simulink model "echo"  (R2020a)
settings: Solver=VariableStepAuto  StartTime=0.0  StopTime=10.0  RelTol=1e-3
libraries: dspspect3 x1, dspvision x1, dspobslib x1
settings Model: Creator=XPS 15  LastModifiedBy=XPS 15

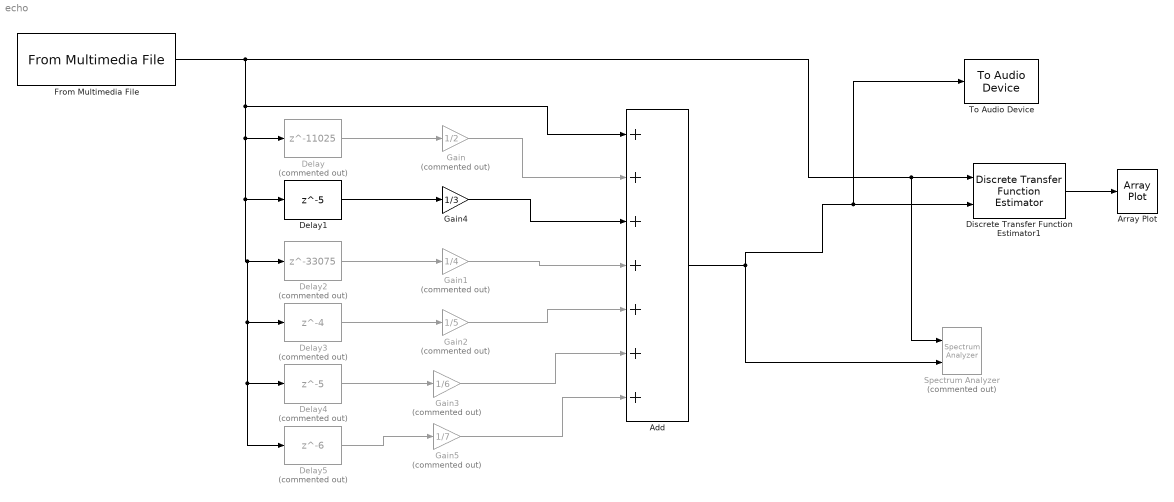
== system echo ==
  Add : Sum  Inputs=+++++++
  Array Plot : ArrayPlot
  Delay : Delay  Commented=on  DelayLength=11025  InitialCondition=0
  Delay1 : Delay  DelayLength=5  InitialCondition=0
  Delay2 : Delay  Commented=on  DelayLength=33075  InitialCondition=0
  Delay3 : Delay  Commented=on  DelayLength=4  InitialCondition=0
  Delay4 : Delay  Commented=on  DelayLength=5  InitialCondition=0
  Delay5 : Delay  Commented=on  DelayLength=6  InitialCondition=0
  Discrete Transfer Function Estimator1 : dspspect3/Discrete Transfer Function Estimator  WindowMode=Specify on dialog  WindowLength=1024  Overlap=50  AveragingMethod=Running  ForgettingFactorPort=off  ForgettingFactor=0.9  SpectralAverages=100  FFTLengthSource=Auto  FFTLength=128  Window=Hann  SidelobeAttenuation=60  FrequencyRange=One-sided  OutputCoherence=off  SimulateUsing=Code generation
      settings: SourceProductBaseCode=DS
  From Multimedia File : dspvision/From Multimedia File  inputFilename=C:\Users\XPS 15\Desktop\L05 Sorbonne\images\Son\Projet\guitare.wav  readRange=[1 Inf]  loop=on  numPlays=inf  outputStreams=Audio only  videoDataType=single  audioDataType=double  inheritSampleTime=on  userDefinedSampleTime=1/30  noAudioOutput=off  isIntensityVideo=off  fourcc=RGB  colorVideoFormat=Separate color signals  outputEOF=off  dataOrg=Column-major  audioFrameSize=1  computeAudioFrameSize=off  outSamplingMode=Sample based
  Gain : Gain  Commented=on  Gain=1/2
  Gain1 : Gain  Commented=on  Gain=1/4
  Gain2 : Gain  Commented=on  Gain=1/5
  Gain3 : Gain  Commented=on  Gain=1/6
  Gain4 : Gain  Gain=1/3
  Gain5 : Gain  Commented=on  Gain=1/7
  Spectrum Analyzer : SpectrumAnalyzer  Commented=on  NumInputPorts=2
  To Audio Device : dspobslib/To Audio Device  deviceName=Default  inheritSampleRate=on  sampleRate=44100  deviceDatatype=Determine from input data type  autoBufferSize=on  bufferSize=4096  queueDuration=1.0  defaultOutputChannelMapping=on  outputChannelMapping=1:2  outputNumUnderrunSamples=off
      settings: SourceProductBaseCode=DS
  wires:
  From Multimedia File/1 -> Add/1, Delay5/1, Delay4/1, Delay3/1, Delay2/1, Delay1/1, Delay/1, Spectrum Analyzer/1, Discrete Transfer Function Estimator1/1
  Add/1 -> Spectrum Analyzer/2, To Audio Device/1, Discrete Transfer Function Estimator1/2
  Gain4/1 -> Add/3
  Discrete Transfer Function Estimator1/1 -> Array Plot/1
  Gain1/1 -> Add/4
  Gain/1 -> Add/2
  Gain2/1 -> Add/5
  Delay/1 -> Gain/1
  Delay1/1 -> Gain4/1
  Delay2/1 -> Gain1/1
  Delay3/1 -> Gain2/1
  Delay4/1 -> Gain3/1
  Gain3/1 -> Add/6
  Delay5/1 -> Gain5/1
  Gain5/1 -> Add/7
